simulink model "Final_de_Cata_simu"  (R2021a)
settings: Solver=VariableStepAuto  StartTime=0.0  StopTime=10  RelTol=1e-3
values from neighbouring files (symbols this model uses):
  A = 10    [Final_de_Cata.m]
  B = -9    [Final_de_Cata.m]
  C = 1    [Final_de_Cata.m]
  D = -1    [Final_de_Cata.m]
  K = acker(A, B, -1)    [Final_de_Cata.m]
  kf = 1    [Final_de_Cata.m]
  ue = u_hat_e    [Final_de_Cata.m]
  xe = [x1e; x2e; x3e]    [Final_de_Cata.m]
  ye = 20    [Final_de_Cata.m]
libraries: cstblocks x1
settings Model: Creator=Santiago  LastModifiedBy=Santiago

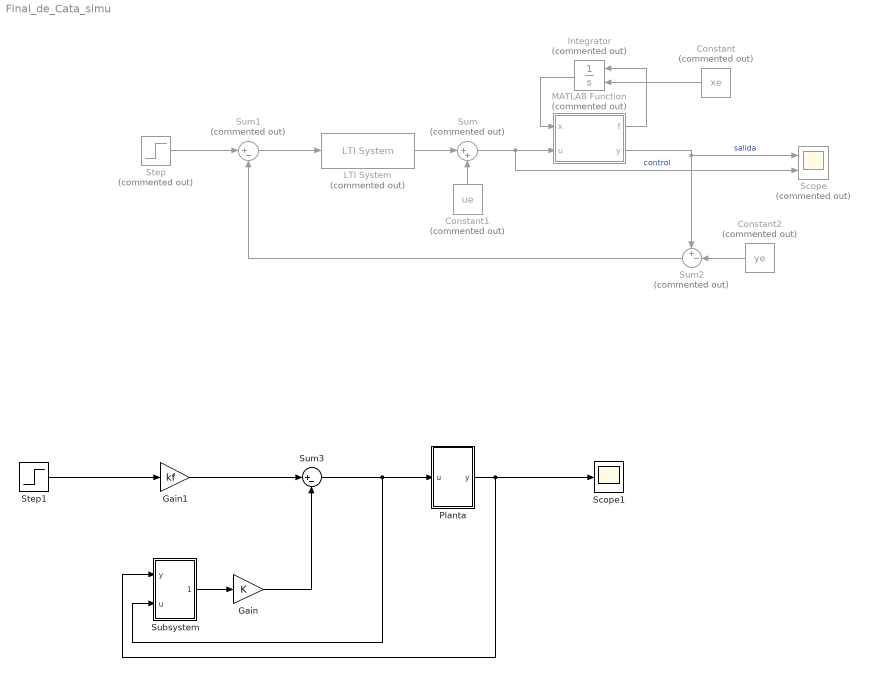
== system Final_de_Cata_simu ==
  Constant : Constant  Commented=on  Value=xe
  Constant1 : Constant  Commented=on  Value=ue
  Constant2 : Constant  Commented=on  Value=ye
  Gain : Gain  Gain=K
  Gain1 : Gain  Gain=kf
  Integrator : Integrator  Commented=on  InitialConditionSource=external
  LTI System : cstblocks/LTI System  Commented=on  sys=C_dig  IC=[]
  MATLAB Function : MATLAB Function  Commented=on  TreatAsAtomicUnit=on
  Planta : Subsystem
  Scope : Scope  Commented=on  NumInputPorts=2
  Scope1 : Scope
  Step : Step  Commented=on  After=4  SampleTime=0
  Step1 : Step  SampleTime=0
  Subsystem : Subsystem
  Sum : Sum  Commented=on  Inputs=|++
  Sum1 : Sum  Commented=on  Inputs=|+-
  Sum2 : Sum  Commented=on  Inputs=+-|
  Sum3 : Sum  Inputs=|+-
  wires:
  MATLAB Function/1(f) -> Integrator/1
  Integrator/1 -> MATLAB Function/1(x)
  Constant/1 -> Integrator/2
  Sum/1 -> Scope/2, MATLAB Function/2(u)  "control"
  LTI System/1 -> Sum/1
  Constant1/1 -> Sum/2
  Sum2/1 -> Sum1/2
  MATLAB Function/2(y) -> Scope/1, Sum2/1  "salida"
  Step/1 -> Sum1/1
  Sum1/1 -> LTI System/1
  Constant2/1 -> Sum2/2
  Subsystem/1(x_est) -> Gain/1
  Gain/1 -> Sum3/2
  Gain1/1 -> Sum3/1
  Sum3/1 -> Subsystem/2(u), Planta/1(u)
  Planta/1(y) -> Scope1/1, Subsystem/1(y)
  Step1/1 -> Gain1/1

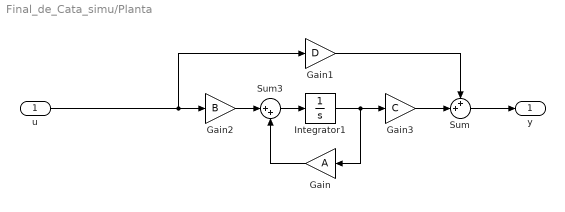
== system Final_de_Cata_simu/Planta ==
  u : Inport
  Gain : Gain  Gain=A
  Gain1 : Gain  Gain=D
  Gain2 : Gain  Gain=B
  Gain3 : Gain  Gain=C
  Integrator1 : Integrator
  Sum : Sum  Inputs=++|
  Sum3 : Sum  Inputs=|++
  y : Outport
  wires:
  Sum3/1 -> Integrator1/1
  Gain2/1 -> Sum3/1
  Gain/1 -> Sum3/2
  Integrator1/1 -> Gain3/1, Gain/1
  u/1 -> Gain1/1, Gain2/1
  Gain3/1 -> Sum/2
  Gain1/1 -> Sum/1
  Sum/1 -> y/1

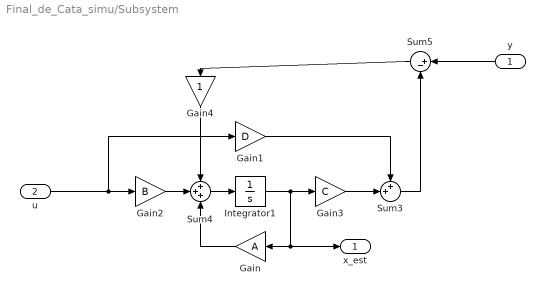
== system Final_de_Cata_simu/Subsystem ==
  y : Inport
  u : Inport  Port=2
  Gain : Gain  Gain=A
  Gain1 : Gain  Gain=D
  Gain2 : Gain  Gain=B
  Gain3 : Gain  Gain=C
  Gain4 : Gain
  Integrator1 : Integrator
  Sum3 : Sum  Inputs=++|
  Sum4 : Sum  Inputs=+++
  Sum5 : Sum  Inputs=|+-
  x_est : Outport
  wires:
  Integrator1/1 -> Gain3/1, x_est/1, Gain/1
  Gain1/1 -> Sum3/1
  Sum3/1 -> Sum5/2
  Sum4/1 -> Integrator1/1
  u/1 -> Gain1/1, Gain2/1
  Gain4/1 -> Sum4/1
  Gain3/1 -> Sum3/2
  Gain/1 -> Sum4/3
  Gain2/1 -> Sum4/2
  Sum5/1 -> Gain4/1
  y/1 -> Sum5/1

== matlab function Final_de_Cata_simu/MATLAB Function ==
  data: x input; f output; u input; y output
function [f, y]  = fcn(x, u)
x1 = x(1);
x2 = x(2);
x3 = x(3);

m = 1600;
alfa4 = 12;
Tm = 190;
beta = 0.4;
wm = 420;
rho = 1.3;
Cd = 0.32;
Af = 2.4;
g = 9.8;
tita = 4 * pi/180;
Cr = 0.01;
wn = 2 * pi;

f1 = alfa4/m * Tm * (1 - beta * (alfa4 / wm * x1 - 1)^2) * x2 - 0.5 * rho/m * Cd * Af * x1^2 - g * sin(tita) - g * Cr;
f2 = x3;
f3 = -wn^2 * x2 - 2 * wn * x3 + wn^2 * u;
f = [f1; f2; f3];

y = x1;
